simulink model "Modele_subsystem"  (R2018b)
settings: Solver=VariableStepAuto  StartTime=0.0  StopTime=10.0  RelTol=1e-3
values from neighbouring files (symbols this model uses):
  ae0 = 1    [Modele.m]
  ae1 = 1    [Modele.m]
  ae2 = 1    [Modele.m]
  ae3 = 1    [Modele.m]
  as0 = 1    [Modele.m]
  as1 = 1    [Modele.m]
  as2 = 1    [Modele.m]
  as3 = 1    [Modele.m]
  be1 = 1    [Modele.m]
  g = 9.81    [Modele.m]
  Js = 2*masseS*Rs^2/5    (= 4.8672e-08)    [Modele.m]
  Jxy = 1347*10^-6    (= 0.001347)    [Modele.m]
  L = 1    [Modele.m]
  masseP = 442/1000    (= 0.442)    [Modele.m]
  masseS = 8/1000    (= 0.008)    [Modele.m]
  R = 1    [Modele.m]
  r_abc = 95.2/1000    (= 0.0952)    [Modele.m]
  Rs = 3.9/1000    (= 0.0039)    [Modele.m]
  XA = r_abc    (= 0.0952)    [Modele.m]
  XB = -r_abc*sind(30)    [Modele.m]
  XC = -r_abc*sind(30)    [Modele.m]
  YA = 0    [Modele.m]
  YB = r_abc*cosd(30)    [Modele.m]
  YC = -r_abc*cosd(30)    [Modele.m]
undefined symbols (not defined in the file or in its folder): La
settings Model: Creator=Vincent  LastModifiedBy=Vincent

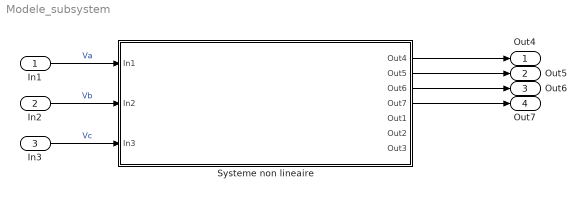
== system Modele_subsystem ==
  In1 : Inport
  In2 : Inport  Port=2
  In3 : Inport  Port=3
  Systeme non lineaire : Subsystem
  Out4 : Outport
  Out5 : Outport  Port=2
  Out6 : Outport  Port=3
  Out7 : Outport  Port=4
  wires:
  In1/1 -> Systeme non lineaire/1(In1)  "Va"
  In2/1 -> Systeme non lineaire/2(In2)  "Vb"
  In3/1 -> Systeme non lineaire/3(In3)  "Vc"
  Systeme non lineaire/1(Out4) -> Out4/1
  Systeme non lineaire/2(Out5) -> Out5/1
  Systeme non lineaire/3(Out6) -> Out6/1
  Systeme non lineaire/4(Out7) -> Out7/1

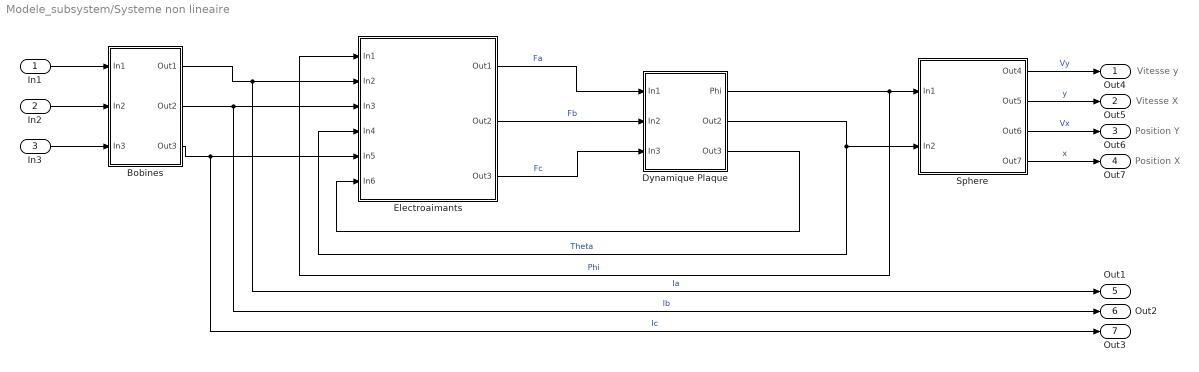
== system Modele_subsystem/Systeme non lineaire ==
  note: Position X
  note: Vitesse X
  note: Position Y
  note: Vitesse y
  In1 : Inport
  In2 : Inport  Port=2
  In3 : Inport  Port=3
  Bobines : Subsystem
  Dynamique Plaque : Subsystem
  Electroaimants : Subsystem
  Sphere : Subsystem
  Out4 : Outport
  Out5 : Outport  Port=2
  Out6 : Outport  Port=3
  Out7 : Outport  Port=4
  Out1 : Outport  Port=5
  Out2 : Outport  Port=6
  Out3 : Outport  Port=7
  wires:
  Electroaimants/2(Out2) -> Dynamique Plaque/2(In2)  "Fb"
  Bobines/2(Out2) -> Out2/1, Electroaimants/3(In3)  "Ib"
  Bobines/1(Out1) -> Out1/1, Electroaimants/2(In2)  "Ia"
  Dynamique Plaque/2(Out2) -> Electroaimants/4(In4), Sphere/2(In2)  "Theta"
  In2/1 -> Bobines/2(In2)
  Electroaimants/1(Out1) -> Dynamique Plaque/1(In1)  "Fa"
  In1/1 -> Bobines/1(In1)
  Electroaimants/3(Out3) -> Dynamique Plaque/3(In3)  "Fc"
  Dynamique Plaque/1(Phi) -> Electroaimants/1(In1), Sphere/1(In1)  "Phi"
  Bobines/3(Out3) -> Out3/1, Electroaimants/5(In5)  "Ic"
  Dynamique Plaque/3(Out3) -> Electroaimants/6(In6)
  In3/1 -> Bobines/3(In3)
  Sphere/1(Out4) -> Out4/1  "Vy"
  Sphere/2(Out5) -> Out5/1  "y"
  Sphere/3(Out6) -> Out6/1  "Vx"
  Sphere/4(Out7) -> Out7/1  "x"

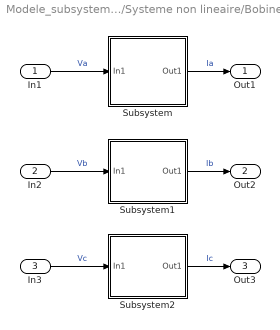
== system Modele_subsystem/Systeme non lineaire/Bobines ==
  In1 : Inport
  In2 : Inport  Port=2
  In3 : Inport  Port=3
  Subsystem : Subsystem
  Subsystem1 : Subsystem
  Subsystem2 : Subsystem
  Out1 : Outport
  Out2 : Outport  Port=2
  Out3 : Outport  Port=3
  wires:
  In1/1 -> Subsystem/1(In1)  "Va"
  In2/1 -> Subsystem1/1(In1)  "Vb"
  Subsystem2/1(Out1) -> Out3/1  "Ic"
  Subsystem/1(Out1) -> Out1/1  "Ia"
  In3/1 -> Subsystem2/1(In1)  "Vc"
  Subsystem1/1(Out1) -> Out2/1  "Ib"

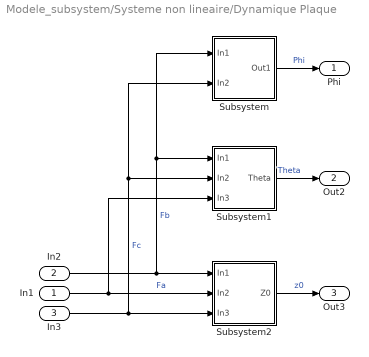
== system Modele_subsystem/Systeme non lineaire/Dynamique Plaque ==
  In1 : Inport
  In2 : Inport  Port=2
  In3 : Inport  Port=3
  Subsystem : Subsystem
  Subsystem1 : Subsystem
  Subsystem2 : Subsystem
  Phi : Outport
  Out2 : Outport  Port=2
  Out3 : Outport  Port=3
  wires:
  In1/1 -> Subsystem1/3(In3), Subsystem2/2(In2)  "Fa"
  In3/1 -> Subsystem/2(In2), Subsystem1/2(In2), Subsystem2/3(In3)  "Fc"
  Subsystem1/1(Theta) -> Out2/1  "Theta"
  In2/1 -> Subsystem1/1(In1), Subsystem/1(In1), Subsystem2/1(In1)  "Fb"
  Subsystem/1(Out1) -> Phi/1  "Phi"
  Subsystem2/1(Z0) -> Out3/1  "z0"

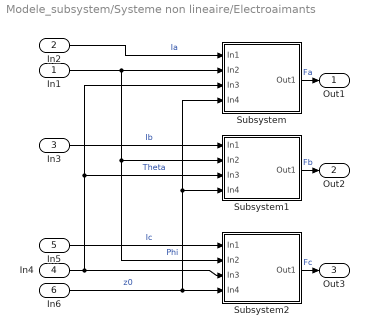
== system Modele_subsystem/Systeme non lineaire/Electroaimants ==
  In1 : Inport
  In2 : Inport  Port=2
  In3 : Inport  Port=3
  In4 : Inport  Port=4
  In5 : Inport  Port=5
  In6 : Inport  Port=6
  Subsystem : Subsystem
  Subsystem1 : Subsystem
  Subsystem2 : Subsystem
  Out1 : Outport
  Out2 : Outport  Port=2
  Out3 : Outport  Port=3
  wires:
  In6/1 -> Subsystem2/4(In4), Subsystem1/4(In4), Subsystem/4(In4)  "z0"
  In4/1 -> Subsystem2/3(In3), Subsystem/3(In3), Subsystem1/3(In3)  "Theta"
  In5/1 -> Subsystem2/1(In1)  "Ic"
  In1/1 -> Subsystem/2(In2), Subsystem2/2(In2), Subsystem1/2(In2)  "Phi"
  Subsystem2/1(Out1) -> Out3/1  "Fc"
  In2/1 -> Subsystem/1(In1)  "Ia"
  In3/1 -> Subsystem1/1(In1)  "Ib"
  Subsystem1/1(Out1) -> Out2/1  "Fb"
  Subsystem/1(Out1) -> Out1/1  "Fa"

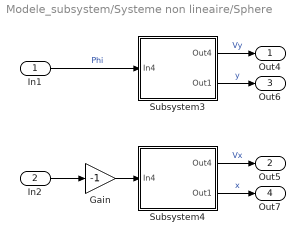
== system Modele_subsystem/Systeme non lineaire/Sphere ==
  In1 : Inport
  In2 : Inport  Port=2
  Gain : Gain  Gain=-1
  Subsystem3 : Subsystem
  Subsystem4 : Subsystem
  Out4 : Outport
  Out5 : Outport  Port=2
  Out6 : Outport  Port=3
  Out7 : Outport  Port=4
  wires:
  Subsystem3/2(Out1) -> Out6/1  "y"
  Subsystem4/1(Out4) -> Out5/1  "Vx"
  Subsystem3/1(Out4) -> Out4/1  "Vy"
  In2/1 -> Gain/1
  Subsystem4/2(Out1) -> Out7/1  "x"
  Gain/1 -> Subsystem4/1(In4)
  In1/1 -> Subsystem3/1(In4)  "Phi"

== system Modele_subsystem/Systeme non lineaire/Bobines/Subsystem ==
  In1 : Inport
  Gain : Gain  Gain=L
  Gain1 : Gain  Gain=R/L
  Integrator : Integrator
  Sum : Sum  Inputs=|+-
  Out1 : Outport
  wires:
  Integrator/1 -> Out1/1, Gain1/1
  Gain/1 -> Sum/1
  Gain1/1 -> Sum/2
  Sum/1 -> Integrator/1
  In1/1 -> Gain/1

== system Modele_subsystem/Systeme non lineaire/Bobines/Subsystem1 ==
  In1 : Inport
  Gain : Gain  Gain=La
  Gain1 : Gain  Gain=R/L
  Integrator : Integrator
  Sum : Sum  Inputs=|+-
  Out1 : Outport
  wires:
  Integrator/1 -> Out1/1, Gain1/1
  Gain/1 -> Sum/1
  Gain1/1 -> Sum/2
  Sum/1 -> Integrator/1
  In1/1 -> Gain/1

== system Modele_subsystem/Systeme non lineaire/Bobines/Subsystem2 ==
  In1 : Inport
  Gain : Gain  Gain=La
  Gain1 : Gain  Gain=R/L
  Integrator : Integrator
  Sum : Sum  Inputs=|+-
  Out1 : Outport
  wires:
  Integrator/1 -> Out1/1, Gain1/1
  Gain/1 -> Sum/1
  Gain1/1 -> Sum/2
  Sum/1 -> Integrator/1
  In1/1 -> Gain/1

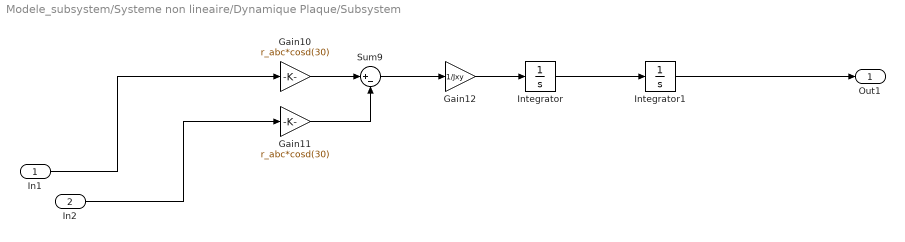
== system Modele_subsystem/Systeme non lineaire/Dynamique Plaque/Subsystem ==
  In1 : Inport
  In2 : Inport  Port=2
  Gain10 : Gain  Gain=r_abc*cosd(30)
  Gain11 : Gain  Gain=r_abc*cosd(30)
  Gain12 : Gain  Gain=1/Jxy
  Integrator : Integrator
  Integrator1 : Integrator
  Sum9 : Sum  Inputs=|+-
  Out1 : Outport
  wires:
  Integrator1/1 -> Out1/1
  In2/1 -> Gain11/1
  Integrator/1 -> Integrator1/1
  Gain10/1 -> Sum9/1
  Sum9/1 -> Gain12/1
  Gain12/1 -> Integrator/1
  Gain11/1 -> Sum9/2
  In1/1 -> Gain10/1

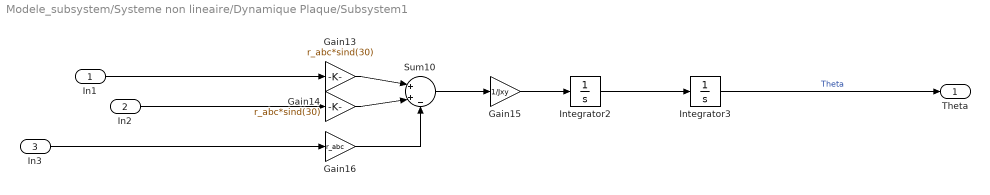
== system Modele_subsystem/Systeme non lineaire/Dynamique Plaque/Subsystem1 ==
  In1 : Inport
  In2 : Inport  Port=2
  In3 : Inport  Port=3
  Gain13 : Gain  Gain=r_abc*sind(30)
  Gain14 : Gain  Gain=r_abc*sind(30)
  Gain15 : Gain  Gain=1/Jxy
  Gain16 : Gain  Gain=r_abc
  Integrator2 : Integrator
  Integrator3 : Integrator
  Sum10 : Sum  Inputs=|++-
  Theta : Outport
  wires:
  In3/1 -> Gain16/1
  Gain14/1 -> Sum10/2
  Gain15/1 -> Integrator2/1
  Sum10/1 -> Gain15/1
  Integrator2/1 -> Integrator3/1
  In1/1 -> Gain13/1
  Gain13/1 -> Sum10/1
  Integrator3/1 -> Theta/1  "Theta"
  Gain16/1 -> Sum10/3
  In2/1 -> Gain14/1

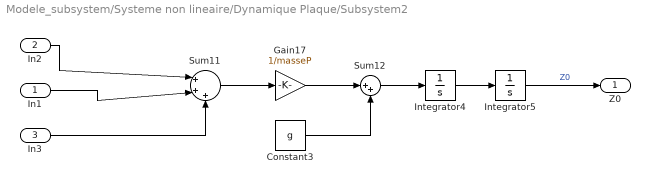
== system Modele_subsystem/Systeme non lineaire/Dynamique Plaque/Subsystem2 ==
  In1 : Inport
  In2 : Inport  Port=2
  In3 : Inport  Port=3
  Constant3 : Constant  Value=g
  Gain17 : Gain  Gain=1/masseP
  Integrator4 : Integrator
  Integrator5 : Integrator
  Sum11 : Sum  Inputs=|+++
  Sum12 : Sum  Inputs=|++
  Z0 : Outport
  wires:
  Integrator5/1 -> Z0/1  "Z0"
  Gain17/1 -> Sum12/1
  In3/1 -> Sum11/3
  Sum11/1 -> Gain17/1
  Constant3/1 -> Sum12/2
  In1/1 -> Sum11/2
  Integrator4/1 -> Integrator5/1
  Sum12/1 -> Integrator4/1
  In2/1 -> Sum11/1

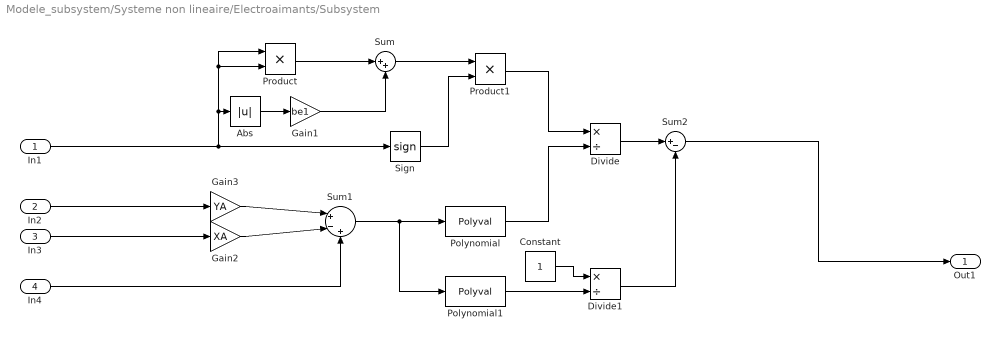
== system Modele_subsystem/Systeme non lineaire/Electroaimants/Subsystem ==
  In1 : Inport
  In2 : Inport  Port=2
  In3 : Inport  Port=3
  In4 : Inport  Port=4
  Abs : Abs
  Constant : Constant
  Divide : Product  Inputs=*/
  Divide1 : Product  Inputs=*/
  Gain1 : Gain  Gain=be1
  Gain2 : Gain  Gain=XA
  Gain3 : Gain  Gain=YA
  Polynomial : Polyval  Coefs=[ae3 ae2 ae1 ae0]
  Polynomial1 : Polyval  Coefs=[as3 as2 as1 as0]
  Product : Product
  Product1 : Product
  Sign : Signum
  Sum : Sum  Inputs=|++
  Sum1 : Sum  Inputs=|+-+
  Sum2 : Sum  Inputs=|+-
  Out1 : Outport
  wires:
  Sum/1 -> Product1/1
  Product1/1 -> Divide/1
  Gain2/1 -> Sum1/2
  Sum2/1 -> Out1/1
  Constant/1 -> Divide1/1
  Product/1 -> Sum/1
  Polynomial/1 -> Divide/2
  In1/1 -> Product/1, Product/2, Abs/1, Sign/1
  Abs/1 -> Gain1/1
  Gain1/1 -> Sum/2
  Polynomial1/1 -> Divide1/2
  Sum1/1 -> Polynomial1/1, Polynomial/1
  Sign/1 -> Product1/2
  In4/1 -> Sum1/3
  Divide/1 -> Sum2/1
  Gain3/1 -> Sum1/1
  Divide1/1 -> Sum2/2
  In2/1 -> Gain3/1
  In3/1 -> Gain2/1

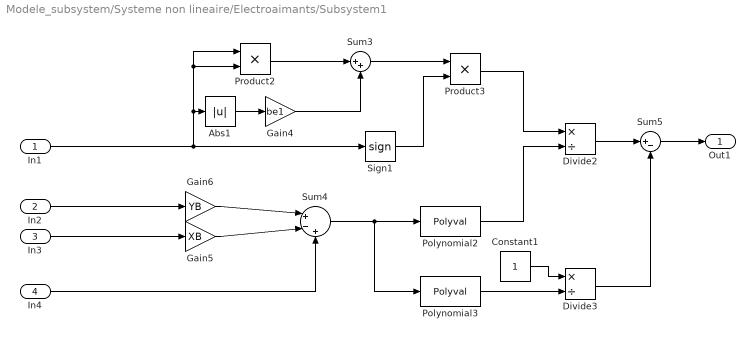
== system Modele_subsystem/Systeme non lineaire/Electroaimants/Subsystem1 ==
  In1 : Inport
  In2 : Inport  Port=2
  In3 : Inport  Port=3
  In4 : Inport  Port=4
  Abs1 : Abs
  Constant1 : Constant
  Divide2 : Product  Inputs=*/
  Divide3 : Product  Inputs=*/
  Gain4 : Gain  Gain=be1
  Gain5 : Gain  Gain=XB
  Gain6 : Gain  Gain=YB
  Polynomial2 : Polyval  Coefs=[ae3 ae2 ae1 ae0]
  Polynomial3 : Polyval  Coefs=[as3 as2 as1 as0]
  Product2 : Product
  Product3 : Product
  Sign1 : Signum
  Sum3 : Sum  Inputs=|++
  Sum4 : Sum  Inputs=|+-+
  Sum5 : Sum  Inputs=|+-
  Out1 : Outport
  wires:
  In2/1 -> Gain6/1
  Gain6/1 -> Sum4/1
  In4/1 -> Sum4/3
  Gain5/1 -> Sum4/2
  Sum4/1 -> Polynomial3/1, Polynomial2/1
  In1/1 -> Product2/1, Product2/2, Abs1/1, Sign1/1
  Constant1/1 -> Divide3/1
  Sign1/1 -> Product3/2
  Divide2/1 -> Sum5/1
  In3/1 -> Gain5/1
  Divide3/1 -> Sum5/2
  Polynomial3/1 -> Divide3/2
  Product3/1 -> Divide2/1
  Gain4/1 -> Sum3/2
  Abs1/1 -> Gain4/1
  Product2/1 -> Sum3/1
  Sum3/1 -> Product3/1
  Polynomial2/1 -> Divide2/2
  Sum5/1 -> Out1/1

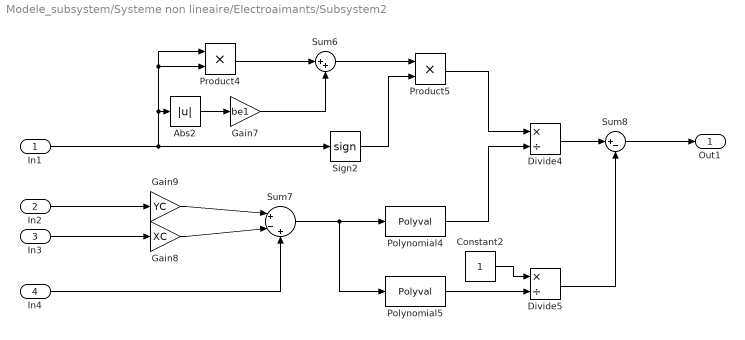
== system Modele_subsystem/Systeme non lineaire/Electroaimants/Subsystem2 ==
  In1 : Inport
  In2 : Inport  Port=2
  In3 : Inport  Port=3
  In4 : Inport  Port=4
  Abs2 : Abs
  Constant2 : Constant
  Divide4 : Product  Inputs=*/
  Divide5 : Product  Inputs=*/
  Gain7 : Gain  Gain=be1
  Gain8 : Gain  Gain=XC
  Gain9 : Gain  Gain=YC
  Polynomial4 : Polyval  Coefs=[ae3 ae2 ae1 ae0]
  Polynomial5 : Polyval  Coefs=[as3 as2 as1 as0]
  Product4 : Product
  Product5 : Product
  Sign2 : Signum
  Sum6 : Sum  Inputs=|++
  Sum7 : Sum  Inputs=|+-+
  Sum8 : Sum  Inputs=|+-
  Out1 : Outport
  wires:
  Gain9/1 -> Sum7/1
  Gain8/1 -> Sum7/2
  Divide5/1 -> Sum8/2
  Divide4/1 -> Sum8/1
  Constant2/1 -> Divide5/1
  In1/1 -> Product4/1, Product4/2, Abs2/1, Sign2/1
  Sum7/1 -> Polynomial5/1, Polynomial4/1
  Sign2/1 -> Product5/2
  In2/1 -> Gain9/1
  Product4/1 -> Sum6/1
  Product5/1 -> Divide4/1
  In4/1 -> Sum7/3
  Polynomial5/1 -> Divide5/2
  Gain7/1 -> Sum6/2
  Polynomial4/1 -> Divide4/2
  Sum6/1 -> Product5/1
  Abs2/1 -> Gain7/1
  Sum8/1 -> Out1/1
  In3/1 -> Gain8/1

== system Modele_subsystem/Systeme non lineaire/Sphere/Subsystem3 ==
  In4 : Inport  Tag=Theta
  Gain : Gain  Gain=masseS*g/(masseS+Js/Rs^2)
  Integrator : Integrator
  Integrator1 : Integrator
  Out4 : Outport
  Out1 : Outport  Port=2
  wires:
  Gain/1 -> Integrator/1
  In4/1 -> Gain/1
  Integrator1/1 -> Out4/1
  Integrator/1 -> Out1/1, Integrator1/1

== system Modele_subsystem/Systeme non lineaire/Sphere/Subsystem4 ==
  In4 : Inport  Tag=Theta
  Gain : Gain  Gain=-masseS*g/(masseS+Js/Rs^2)
  Integrator : Integrator
  Integrator1 : Integrator
  Out4 : Outport
  Out1 : Outport  Port=2
  wires:
  Gain/1 -> Integrator/1
  In4/1 -> Gain/1
  Integrator1/1 -> Out4/1
  Integrator/1 -> Out1/1, Integrator1/1
